simulink model "stateflowmodel"  (R2017a)
settings: Solver=FixedStepDiscrete  StartTime=0.0  StopTime=2900  FixedStep=1  RelTol=1e-3
undefined symbols (not defined in the file): DiscIntNeverNeededParam
settings Model: Creator=hutong  LastModifiedBy=hutong
settings SolverCC: AutoInsertRateTranBlk=on
settings DataIOCC: LimitDataPoints=on
settings OptimizationCC: DefaultParameterBehavior=Inlined  UseDivisionForNetSlopeComputation=on  UseFloatMulNetSlope=on  InlineInvariantSignals=on  PassReuseOutputArgsAs=Individual arguments  ZeroExternalMemoryAtStartup=off  ZeroInternalMemoryAtStartup=off  NoFixptDivByZeroProtection=on  EfficientFloat2IntCast=on  LifeSpan=1
settings DebuggingCC: UnderspecifiedInitializationDetection=Classic  MergeDetectMultiDrivingBlocksExec=none  ParameterTunabilityLossMsg=error  AllowSymbolicDim=off  SFUnexpectedBacktrackingDiag=warning  SFNoUnconditionalDefaultTransitionDiag=warning  SFExecutionAtInitializationDiag=none
settings HardwareCC: ProdBitPerPointer=32  ProdBitPerSizeT=32  ProdBitPerPtrDiffT=32  ProdLargestAtomicInteger=Long  ProdLargestAtomicFloat=Double  ProdWordSize=32  ProdHWDeviceType=ARM Compatible->ARM Cortex
settings SFSimCC: MATLABDynamicMemAlloc=off
settings RTWCC: SystemTargetFile=ert.tlc  TemplateMakefile=ert_default_tmf  Description=Embedded Coder  GenerateReport=on  IncludeHyperlinkInReport=on  LaunchReport=on  GenerateTraceInfo=on  GenerateTraceReport=on  GenerateTraceReportSl=on  GenerateTraceReportSf=on  GenerateTraceReportEml=on  GenerateCodeMetricsReport=on
settings CodeAppCC: ForceParamTrailComments=on  IgnoreCustomStorageClasses=off  OperatorAnnotations=on  SimulinkDataObjDesc=on  SFDataObjDesc=on  MATLABFcnDesc=on  CustomSymbolStrGlobalVar=rt$N$M  CustomSymbolStrType=$N$M  CustomSymbolStrFcn=$N$M$F  CustomSymbolStrMacro=$N$M  InsertBlockDesc=on  MATLABSourceComments=on
settings ERTTargetCC: GenerateSampleERTMain=on  IncludeMdlTerminateFcn=off  CombineSignalStateStructs=on  SupportComplex=off  SupportNonInlinedSFcns=on  InlinedParameterPlacement=NonHierarchical  ERTCustomFileTemplate=example_file_process.tlc  ERTFilePackagingFormat=CompactWithDataFile
settings ConfigComp: CovMetricSettings=dw  CovHtmlReporting=on  CovSaveCumulativeToWorkspaceVar=on  CovSaveSingleToWorkspaceVar=on  CovShowResultsExplorer=off  CovExternalEMLEnable=off  CovSFcnEnable=off

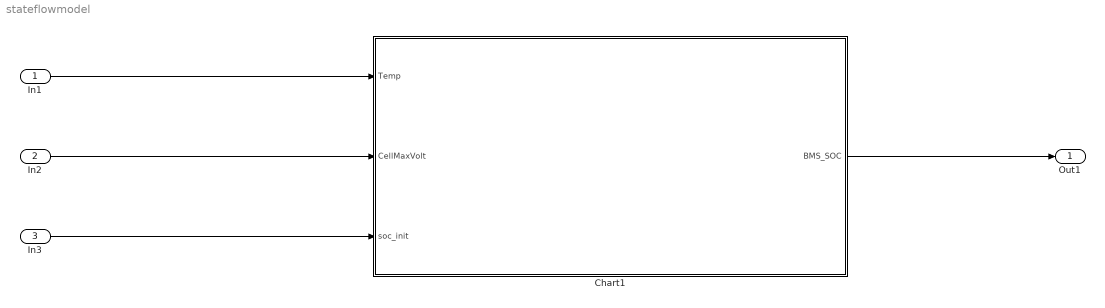
== system stateflowmodel ==
  In1 : Inport
  In2 : Inport  Port=2
  In3 : Inport  Port=3
  Chart1 : Stateflow chart  TreatAsAtomicUnit=on
  Out1 : Outport
  wires:
  Chart1/1(BMS_SOC) -> Out1/1
  In1/1 -> Chart1/1(Temp)
  In2/1 -> Chart1/2(CellMaxVolt)
  In3/1 -> Chart1/3(soc_init)

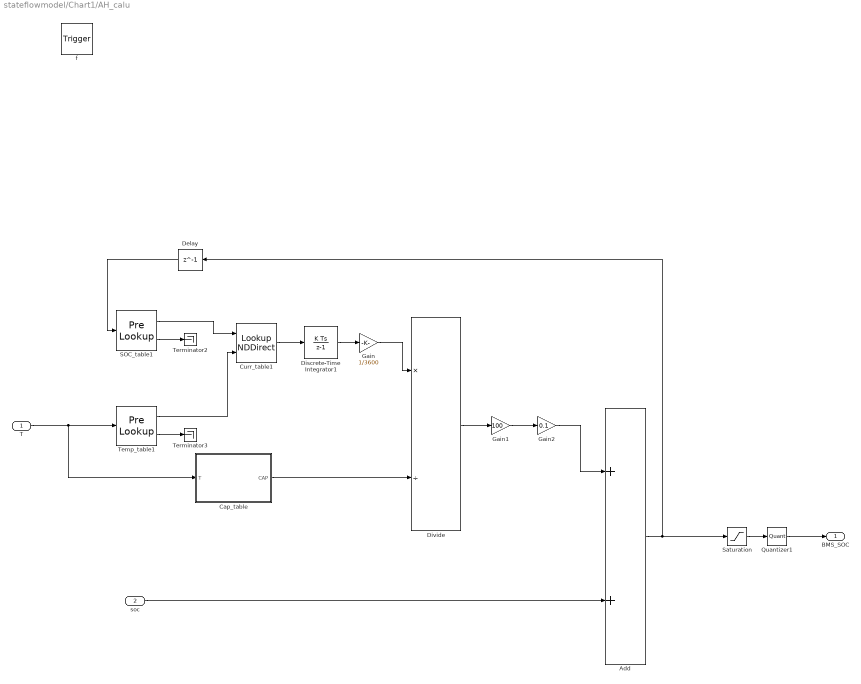
== system stateflowmodel/Chart1/AH_calu ==
  T : Inport  OutDataTypeStr=double  PortDimensions=[1 1]
  soc : Inport  Port=2  OutDataTypeStr=double  PortDimensions=[1 1]
  f : TriggerPort  TriggerType=function-call  VariantControl=Variant
      settings: CopyFcn=Stateflow.SLINSF.SimulinkMan.removeBlockPreDeleteFcn  PreDeleteFcn=Stateflow.SLINSF.SimulinkMan.unsafePredeleteFcn
  Add : Sum
  Cap_table : MATLAB Function  TreatAsAtomicUnit=on
  Curr_table1 : LookupNDDirect  Table=reshape([0,0,0,0,0,0,0,0,0,0,0,0,7,7,18,18,14,14,14,7,7,7,7,7,7,18,28,28,18,18,18,18,18,18,7,7,14,42,71,71,42,42,42,42,42,18,7,7,14,42,113,113,85,71,71,71,42,28,28,14,28,71,142,142,113,113,113,113,113,28,28,14,28,71,170,170,142,142,142,113,113,71,42,28,28,71,170,170,142,142,142,113,113,71,42,28,28,71,170,170,142,142,142,113,113,71,42,28,28,56,113,113,85,85,85,85,85,56,56,28,28,42,85,85,71,71,56,56,42,28,28,14,28,42,85,85,71,71,56,56,42,28,28,14,28,28,56,56,42,42,28,28,28,14,14,7],12,13)
  Delay : Delay  DelayLength=1  InitialCondition=0
  Discrete-Time Integrator1 : DiscreteIntegrator  gainval=1  InitialConditionSetting=State (most efficient)  SampleTime=-1  ICPrevOutput=DiscIntNeverNeededParam  ICPrevScaledInput=DiscIntNeverNeededParam
  Divide : Product  Inputs=*/
  Gain : Gain  Gain=1/3600
  Gain1 : Gain  Gain=100
  Gain2 : Gain  Gain=0.1
  Quantizer1 : Quantizer  QuantizationInterval=0.1
  SOC_table1 : PreLookup  BreakpointsData=[0,5,[10:10:90],95,100]  ExtrapMethod=Linear
  Saturation : Saturate  UpperLimit=100  LowerLimit=0
  Temp_table1 : PreLookup  BreakpointsData=[-30,[0:5:50],52,55]  ExtrapMethod=Linear
  Terminator2 : Terminator
  Terminator3 : Terminator
  BMS_SOC : Outport
  wires:
  Curr_table1/1 -> Discrete-Time Integrator1/1
  SOC_table1/1 -> Curr_table1/1
  Saturation/1 -> Quantizer1/1
  SOC_table1/2 -> Terminator2/1
  Temp_table1/1 -> Curr_table1/2
  Discrete-Time Integrator1/1 -> Gain/1
  Gain/1 -> Divide/1
  Temp_table1/2 -> Terminator3/1
  Cap_table/1(CAP) -> Divide/2
  Divide/1 -> Gain1/1
  T/1 -> Cap_table/1(T), Temp_table1/1
  Delay/1 -> SOC_table1/1
  Gain1/1 -> Gain2/1
  Gain2/1 -> Add/1
  soc/1 -> Add/2
  Add/1 -> Saturation/1, Delay/1
  Quantizer1/1 -> BMS_SOC/1

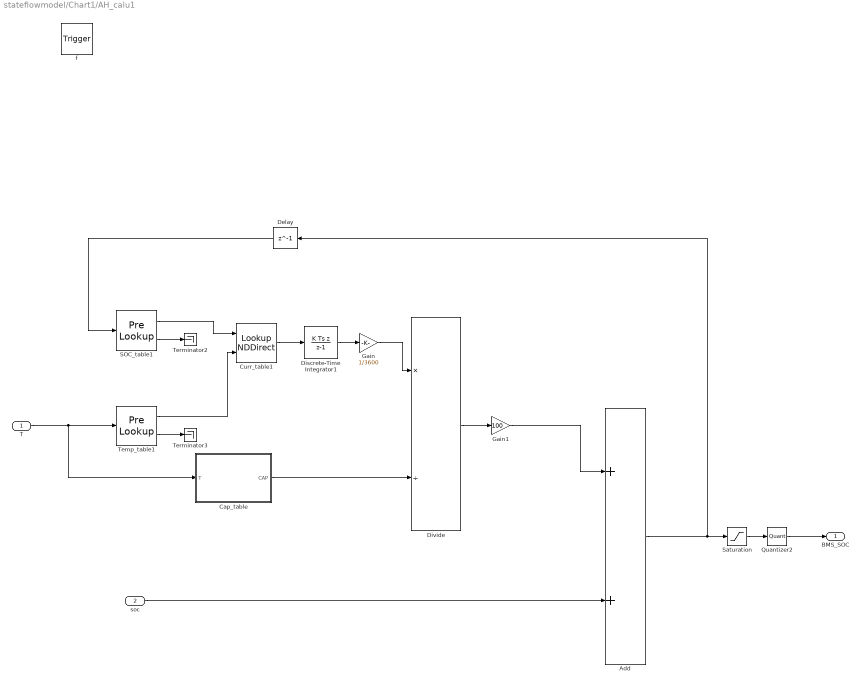
== system stateflowmodel/Chart1/AH_calu1 ==
  T : Inport  OutDataTypeStr=double  PortDimensions=[1 1]
  soc : Inport  Port=2  OutDataTypeStr=double  PortDimensions=[1 1]
  f : TriggerPort  TriggerType=function-call  VariantControl=Variant
      settings: CopyFcn=Stateflow.SLINSF.SimulinkMan.removeBlockPreDeleteFcn  PreDeleteFcn=Stateflow.SLINSF.SimulinkMan.unsafePredeleteFcn
  Add : Sum
  Cap_table : MATLAB Function  TreatAsAtomicUnit=on
  Curr_table1 : LookupNDDirect  Table=|
      | [0 7 7 14 14 28 28 28 28 28 28 28 28
      | ;0	7	18	42	42	71	71	71	71	56	42	42	28;0	18	28	71	113	142	170	170	170	113	85	85	56
      | ;0	18	28	71	113	142	170	170	170	113	85	85	56
      | ;0	14	18	42	85	113	142	142	142	85	71	71	42
      | ;0	14	18	42	71	113	142	142	142	85	71	71	42
      | ;0	14	18	42	71	113	142	142	142	85	56	56	28
      | ;0	7	18	42	71	113	113	113	113	85	56	56	28
      | ;0	7	18	42	71	113	113	113	113	85	42	42	28
      | ;0	7	18	18	28	28	71	71	71	56	28	28	14
      | ;0	7	7	7	28	28	42	42	42	56	28	28	14
      | ;0	7	7	7	14	14	28	28	28	28	14	14	7
      | ]
  Delay : Delay  DelayLength=1  InitialCondition=0
  Discrete-Time Integrator1 : DiscreteIntegrator  IntegratorMethod=Integration: Backward Euler  gainval=1  SampleTime=-1  ICPrevOutput=DiscIntNeverNeededParam  ICPrevScaledInput=DiscIntNeverNeededParam
  Divide : Product  Inputs=*/
  Gain : Gain  Gain=1/3600
  Gain1 : Gain  Gain=100
  Quantizer2 : Quantizer  QuantizationInterval=0.1
  SOC_table1 : PreLookup  BreakpointsData=[0,5,[10:10:90],95,100]  ExtrapMethod=Linear
  Saturation : Saturate  UpperLimit=100  LowerLimit=0
  Temp_table1 : PreLookup  BreakpointsData=[-30,[0:5:50],52,55]  ExtrapMethod=Linear
  Terminator2 : Terminator
  Terminator3 : Terminator
  BMS_SOC : Outport
  wires:
  Curr_table1/1 -> Discrete-Time Integrator1/1
  SOC_table1/1 -> Curr_table1/1
  Saturation/1 -> Quantizer2/1
  SOC_table1/2 -> Terminator2/1
  Temp_table1/1 -> Curr_table1/2
  Discrete-Time Integrator1/1 -> Gain/1
  Gain/1 -> Divide/1
  Temp_table1/2 -> Terminator3/1
  Cap_table/1(CAP) -> Divide/2
  T/1 -> Cap_table/1(T), Temp_table1/1
  Gain1/1 -> Add/1
  soc/1 -> Add/2
  Add/1 -> Delay/1, Saturation/1
  Divide/1 -> Gain1/1
  Quantizer2/1 -> BMS_SOC/1
  Delay/1 -> SOC_table1/1

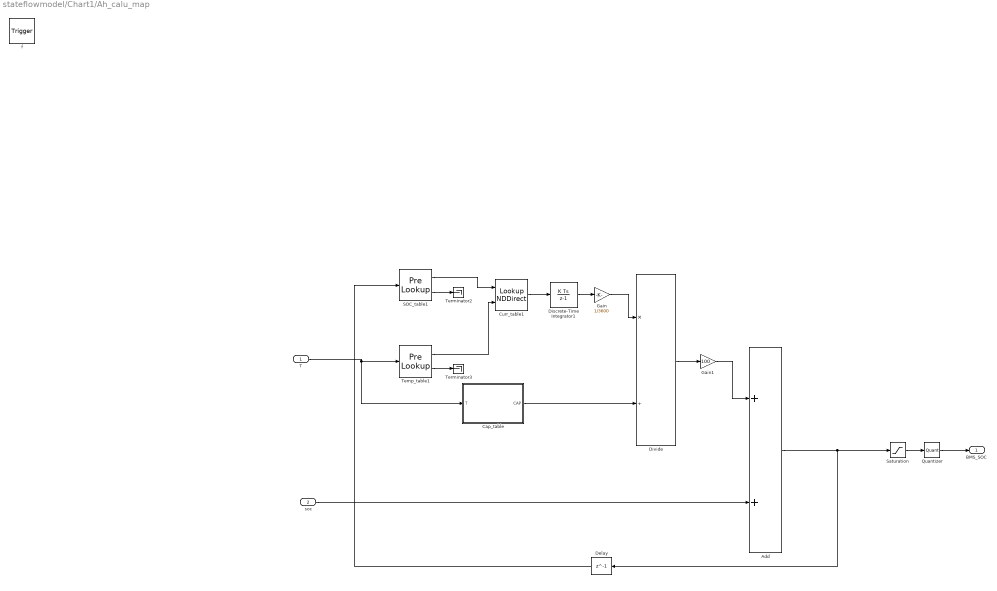
== system stateflowmodel/Chart1/Ah_calu_map ==
  T : Inport  OutDataTypeStr=double  PortDimensions=[1 1]
  soc : Inport  Port=2  OutDataTypeStr=double  PortDimensions=[1 1]
  f : TriggerPort  TriggerType=function-call  VariantControl=Variant
      settings: CopyFcn=Stateflow.SLINSF.SimulinkMan.removeBlockPreDeleteFcn  PreDeleteFcn=Stateflow.SLINSF.SimulinkMan.unsafePredeleteFcn
  Add : Sum
  Cap_table : MATLAB Function  TreatAsAtomicUnit=on
  Curr_table1 : LookupNDDirect  Table=reshape([0,0,0,0,0,0,0,0,0,0,0,0,7,7,18,18,14,14,14,7,7,7,7,7,7,18,28,28,18,18,18,18,18,18,7,7,14,42,71,71,42,42,42,42,42,18,7,7,14,42,113,113,85,71,71,71,42,28,28,14,28,71,142,142,113,113,113,113,113,28,28,14,28,71,170,170,142,142,142,113,113,71,41,28,28,71,170,170,142,142,142,113,113,71,41,28,28,71,170,170,142,142,142,113,113,71,41,28,28,56,113,113,85,85,85,85,85,56,56,28,28,42,85,85,71,71,56,56,42,28,28,14,28,42,85,85,71,71,56,56,42,28,28,14,28,28,56,56,42,42,28,28,28,14,14,7],12,13)  DiagnosticForOutOfRangeInput=None
  Delay : Delay  DelayLength=1  InitialCondition=0
  Discrete-Time Integrator1 : DiscreteIntegrator  InitialConditionSetting=State (most efficient)  SampleTime=-1  ICPrevOutput=DiscIntNeverNeededParam  ICPrevScaledInput=DiscIntNeverNeededParam
  Divide : Product  Inputs=*/
  Gain : Gain  Gain=1/3600
  Gain1 : Gain  Gain=100
  Quantizer : Quantizer  QuantizationInterval=0.1
  SOC_table1 : PreLookup  BreakpointsData=[0,5,[10:10:90],95,100]  ExtrapMethod=Linear
  Saturation : Saturate  UpperLimit=100  LowerLimit=0
  Temp_table1 : PreLookup  BreakpointsData=[-30,[0:5:50],52,55]  ExtrapMethod=Linear
  Terminator2 : Terminator
  Terminator3 : Terminator
  BMS_SOC : Outport
  wires:
  Curr_table1/1 -> Discrete-Time Integrator1/1
  Discrete-Time Integrator1/1 -> Gain/1
  T/1 -> Cap_table/1(T), Temp_table1/1
  Gain/1 -> Divide/1
  Temp_table1/2 -> Terminator3/1
  Cap_table/1(CAP) -> Divide/2
  Add/1 -> Delay/1, Saturation/1
  Divide/1 -> Gain1/1
  soc/1 -> Add/2
  SOC_table1/2 -> Terminator2/1
  SOC_table1/1 -> Curr_table1/1
  Temp_table1/1 -> Curr_table1/2
  Gain1/1 -> Add/1
  Saturation/1 -> Quantizer/1
  Quantizer/1 -> BMS_SOC/1
  Delay/1 -> SOC_table1/1

== stateflow chart stateflowmodel/Chart1 ==
  state Correct91_0_1Ah
    du:
    BMS_SOC =AH_calu(Temp,91);
    temp_soc=AH_calu(Temp,91);
  state Init
    en:
    BMS_SOC=soc_init;
    du:
    BMS_SOC=Ah_calu_map(Temp,soc_init );
  state Correct94_1_Ah
    du:
    BMS_SOC=AH_calu1(Temp,94)
  state Correct91_1_Ah
    en:
    BMS_SOC=temp_soc;
    du:
    BMS_SOC=AH_calu1(Temp,temp_soc)
  state BMS_SOC = AH_calu1(T,soc) [function]
  state BMS_SOC = AH_calu(T,soc) [function]
  state Correct100_soc
    du:
    BMS_SOC=100;
  state BMS_SOC = Ah_calu_map(T,soc) [function]
  Init -> Correct91_0_1Ah [order 2] : [BMS_SOC>=91&&CellMaxVolt<3.413]
  (default) -> Init
  Correct91_0_1Ah -> Correct100_soc [order 2] : [CellMaxVolt>=3.65]
  Correct91_0_1Ah -> Correct91_1_Ah [order 1] : [CellMaxVolt>=3.413]
  Init -> Correct100_soc [order 1] : [CellMaxVolt>=3.65]
  Correct91_1_Ah -> Correct94_1_Ah : [CellMaxVolt>=3.417]
  Correct94_1_Ah -> Correct100_soc : [CellMaxVolt>=3.65]
  data: T function_input double size=[1 1]; BMS_SOC function_output; soc function_input double size=[1 1]; T function_input double size=[1 1]; BMS_SOC function_output; soc function_input double size=[1 1]; T function_input double size=[1 1]; BMS_SOC function_output; soc function_input double size=[1 1]; BMS_SOC output; Temp input; CellMaxVolt input; soc_init input; temp_soc local double

== matlab function stateflowmodel/Chart1/AH_calu/Cap_table ==
  data: T input; CAP output
function CAP = fcn(T)
t=[-30,-20,-10,0,10,25,45,55];
CapPercent=[70,80,85,90,92,100,99,99];
cap=142;
for i = 1:8
    if T == t(i)
        CAP = CapPercent(i)*0.01*cap;
        return;
    else
        if T>t(i)&&T<t(i+1)
            CAP=(0.1*(CapPercent(i+1)-CapPercent(i))*(T-t(i))+CapPercent(i))*0.01*cap;
            return;
        else
            CAP =-1;
        end
    end
end

== matlab function stateflowmodel/Chart1/AH_calu1/Cap_table ==
  data: T input; CAP output
function CAP = fcn(T)
t=[-30,-20,-10,0,10,25,45,55];
CapPercent=[70,80,85,90,92,100,99,99];
cap=142;
for i = 1:8
    if T == t(i)
        CAP = CapPercent(i)*0.01*cap;
        return;
    else
        if T>t(i)&&T<t(i+1)
            CAP=(0.1*(CapPercent(i+1)-CapPercent(i))*(T-t(i))+CapPercent(i))*0.01*cap;
            return;
        else
            CAP =-1;
        end
    end
end

== matlab function stateflowmodel/Chart1/Ah_calu_map/Cap_table ==
  data: T input; CAP output
function CAP = fcn(T)
t=[-30,-20,-10,0,10,25,45,55];
CapPercent=[70,80,85,90,92,100,99,99];
cap=142;
for i = 1:8
    if T == t(i)
        CAP = CapPercent(i)*0.01*cap;
        return;
    else
        if T>t(i)&&T<t(i+1)
            CAP=(0.1*(CapPercent(i+1)-CapPercent(i))*(T-t(i))+CapPercent(i))*0.01*cap;
            return;
        else
            CAP =-1;
        end
    end
end
